simulink model "untitled"  (R2023a)
settings: Solver=VariableStepAuto  StartTime=0.0  StopTime=1  FixedStep=1e-7  MaxStep=2e-7  RelTol=1e-4
model workspace (MAT data in the model file):
  Cout = 0.00069
  Cout_esr = 0.02
  Iout_user_max = 5
  Ki_i = 800
  Ki_v = 30
  Kp_i = 0.025
  Kp_v = 0.2
  L_dcr = 0.02
  L_power = 2.2e-05
  Pout_max = 90
  Rload_extra = 8.57142857143
  Rload_heavy = 6
  Rload_light = 20
  Ts_i = 1e-05
  Ts_v = 0.0001
  Vin = 20
  Vref_max = 30
  Vref_min = 0.5
  Vset = 12
  fsw = 100000
  tdead = 2e-07
libraries: spsSeriesRLCBranchLib x4, spsMosfetLib x4, spsCurrentMeasurementLib x2, eePwmGenerator x2, spsDCVoltageSourceLib x1, spsIdealSwitchLib x1, spsMultimeterLib x1, spsVoltageMeasurementLib x1, spspowerguiLib x1
settings Model: SimulationMode=rapid-accelerator  Creator=39826  LastModifiedBy=39826

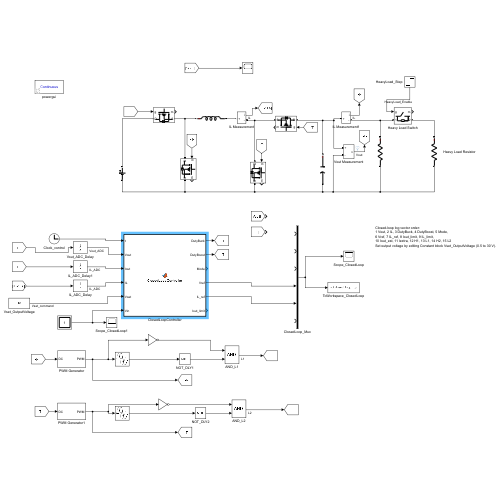
[thumbnail: Simulink's stored preview of the top-level diagram]
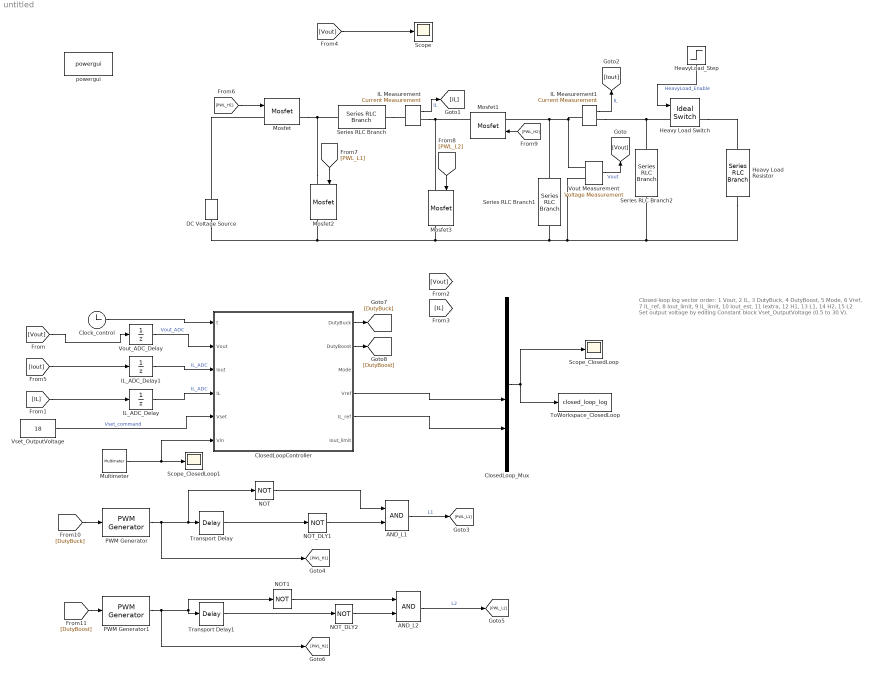
== system untitled ==
  note: Closed-loop log vector order:
      | 1 Vout, 2 IL, 3 DutyBuck, 4 DutyBoost, 5 Mode,
      | 6 Vref, 7 IL_ref, 8 Iout_limit, 9 IL_limit,
      | 10 Iout_est, 11 Iextra, 12 H1, 13 L1, 14 H2, 15 L2
      | Set output voltage by editing Constant block Vset_OutputVoltage (0.5 to 30 V).
  AND_L1 : Logic  AllPortsSameDT=off  OutDataTypeStr=boolean
  AND_L2 : Logic  AllPortsSameDT=off  OutDataTypeStr=boolean
  Clock_control : Clock
  ClosedLoopController : MATLAB Function  TreatAsAtomicUnit=on
  ClosedLoop_Mux : Mux  Inputs=6
  DC Voltage Source : spsDCVoltageSourceLib/DC Voltage Source  Amplitude=Vin  Measurements=Voltage
  Heavy Load Resistor : spsSeriesRLCBranchLib/Series RLC Branch  LConnTagsString=__new0  RConnTagsString=__new0  BranchType=R  Resistance=Rload_extra  Inductance=1e-3  SetiL0=off  InitialCurrent=0  Capacitance=1e-6  Setx0=off  InitialVoltage=0  Measurements=Branch voltage and current
  Heavy Load Switch : spsIdealSwitchLib/Ideal Switch  Ron=3e-3  Lon=0  IC=0  Rs=1e6  Cs=inf  Measurements=on
  HeavyLoad_Step : Step  SampleTime=0
  IL Measurement : spsCurrentMeasurementLib/Current Measurement  PhasorSimulation=off  OutputType=Complex  PSBequivalent=0
  IL Measurement1 : spsCurrentMeasurementLib/Current Measurement  PhasorSimulation=off  OutputType=Complex  PSBequivalent=0
  IL_ADC_Delay : UnitDelay  SampleTime=1e-6  HasFrameUpgradeWarning=on
  IL_ADC_Delay1 : UnitDelay  SampleTime=1e-6  HasFrameUpgradeWarning=on
  Mosfet{,1..3} (4 alike) : spsMosfetLib/Mosfet  Ron=3e-3  Lon=0  Rd=0.01  Vfd=0  IC=0  Rs=1e5  Cs=inf  Measurements=on
  Multimeter : spsMultimeterLib/Multimeter  L=9  sel=5  yselected={}  Gain=1  OutputType=Complex  PlotAtSimulationStop=off  PhasorSimulation=off
  NOT : Logic  Operator=NOT  IconShape=distinctive  AllPortsSameDT=off  OutDataTypeStr=boolean
  NOT1 : Logic  Operator=NOT  IconShape=distinctive  AllPortsSameDT=off  OutDataTypeStr=boolean
  NOT_DLY1 : Logic  Operator=NOT  AllPortsSameDT=off  OutDataTypeStr=boolean
  NOT_DLY2 : Logic  Operator=NOT  AllPortsSameDT=off  OutDataTypeStr=boolean
  PWM Generator : eePwmGenerator/PWM Generator  CarrCount=Up  Tper=1e-5  Tdelay=0  Ts=0
  PWM Generator1 : eePwmGenerator/PWM Generator  CarrCount=Up  Tper=1e-5  Tdelay=0  Ts=0
  Scope : Scope
  Scope_ClosedLoop : Scope
  Scope_ClosedLoop1 : Scope
  Series RLC Branch : spsSeriesRLCBranchLib/Series RLC Branch  LConnTagsString=__new0  RConnTagsString=__new0  BranchType=L  Resistance=L_dcr  Inductance=L_power  SetiL0=off  InitialCurrent=0  Capacitance=1e-6  Setx0=off  InitialVoltage=0  Measurements=Branch voltage and current
  Series RLC Branch1 : spsSeriesRLCBranchLib/Series RLC Branch  LConnTagsString=__new0  RConnTagsString=__new0  BranchType=C  Resistance=Cout_esr  Inductance=1e-3  SetiL0=off  InitialCurrent=0  Capacitance=Cout  Setx0=off  InitialVoltage=0  Measurements=Branch voltage and current
  Series RLC Branch2 : spsSeriesRLCBranchLib/Series RLC Branch  LConnTagsString=__new0  RConnTagsString=__new0  BranchType=R  Resistance=Rload_light  Inductance=1e-3  SetiL0=off  InitialCurrent=0  Capacitance=1e-6  Setx0=off  InitialVoltage=0  Measurements=Branch voltage and current
  ToWorkspace_ClosedLoop : ToWorkspace  VariableName=closed_loop_log  SaveFormat=Structure With Time  SampleTime=-1
  Transport Delay : TransportDelay  DelayTime=tdead
  Transport Delay1 : TransportDelay  DelayTime=tdead
  Vout Measurement : spsVoltageMeasurementLib/Voltage Measurement  PhasorSimulation=off  OutputType=Complex  PSBequivalent=0
  Vout_ADC_Delay : UnitDelay  SampleTime=1e-6  HasFrameUpgradeWarning=on
  Vset_OutputVoltage : Constant  Value=18
  powergui : spspowerguiLib/powergui  Priority=1  SimulationMode=Continuous  SampleTime=1e-7  frequency=60  Iterations=50  frequencyindice=0  Pbase=100e6  ErrMax=1e-4  UnitsV=kV  UnitsW=MW  buscounter=0  FunctionMessages=off  echomessages=off  EnableUseOfTLC=off  CurrentSourceSwitches=off  DisableSnubberDevices=off  DisableRonSwitches=off  DisableVfSwitches=off  DisplayEquations=off  AutomaticDiscreteSolvers=off  SolverType=Tustin/Backward Euler (TBE)  Interpol=off  ExternalGateDelay=off  methode=off  Ts=100  x0status=blocks  SPID=on  SwTol=0  HookPort=off  NonlinearTolerance=1e-4  nMaxIteration=100  ContinueOnMaxIteration=off  RestoreLinks=warning  ResistiveCurrentMeasurement=off  Frange=[0:2:500]  Ylog=off  Xlog=on  ShowGrid=off  save=off  variable=ZData  structure=0  ZoomFFT=off  StartTime=0.0  cycles=1  DisplayStyle=1  fundamental=60  FreqAxis=off  MaxFrequency=1000  frequencyindicesteady=1  RmsSteady=1  display=off
  wires:
  HeavyLoad_Step/1 -> Heavy Load Switch/1  "HeavyLoad_Enable"
  Clock_control/1 -> ClosedLoopController/1(t)
  Vout_ADC_Delay/1 -> ClosedLoopController/2(Vout)  "Vout_ADC"
  Vset_OutputVoltage/1 -> ClosedLoopController/5(Vset)  "Vset_command"
  ClosedLoop_Mux/1 -> Scope_ClosedLoop/1, ToWorkspace_ClosedLoop/1
  Vout Measurement/1 -> [Vout]  "Vout"
  [Vout] -> Vout_ADC_Delay/1
  IL Measurement/1 -> [IL]  "IL"
  [IL] -> IL_ADC_Delay/1
  [Vout] -> Scope/1
  IL_ADC_Delay/1 -> ClosedLoopController/4(IL)  "IL_ADC"
  IL Measurement1/1 -> [Iout]  "IL"
  [Iout] -> IL_ADC_Delay1/1
  IL_ADC_Delay1/1 -> ClosedLoopController/3(Iout)  "IL_ADC"
  Multimeter/1 -> Scope_ClosedLoop1/1, ClosedLoopController/6(Vin)
  PWM Generator/1 -> NOT/1, Transport Delay/1, [PWL_H1]
  PWM Generator1/1 -> NOT1/1, Transport Delay1/1, [PWL_H2]
  [PWL_H1] -> Mosfet/1
  [PWL_L1] -> Mosfet2/1
  [PWL_L2] -> Mosfet3/1
  [PWL_H2] -> Mosfet1/1
  ClosedLoopController/1(DutyBuck) -> [DutyBuck]
  ClosedLoopController/2(DutyBoost) -> [DutyBoost]
  [DutyBuck] -> PWM Generator/1
  [DutyBoost] -> PWM Generator1/1
  ClosedLoopController/5(IL_ref) -> ClosedLoop_Mux/5
  ClosedLoopController/4(Vref) -> ClosedLoop_Mux/4
  Transport Delay/1 -> NOT_DLY1/1
  NOT/1 -> AND_L1/1
  NOT_DLY1/1 -> AND_L1/2
  AND_L1/1 -> [PWL_L1]  "L1"
  Transport Delay1/1 -> NOT_DLY2/1
  NOT1/1 -> AND_L2/1
  NOT_DLY2/1 -> AND_L2/2
  AND_L2/1 -> [PWL_L2]  "L2"
  connections:
  Mosfet/LConn1 -- DC Voltage Source/RConn1
  Mosfet2/LConn1 -- Series RLC Branch/LConn1 -- Mosfet/RConn1
  Series RLC Branch/RConn1 -- IL Measurement/LConn1
  Mosfet3/LConn1 -- Mosfet1/RConn1 -- IL Measurement/RConn1
  Mosfet2/RConn1 -- DC Voltage Source/LConn1 -- Vout Measurement/LConn2 -- Heavy Load Resistor/RConn1 -- Series RLC Branch2/RConn1 -- Series RLC Branch1/RConn1 -- Mosfet3/RConn1
  Series RLC Branch2/LConn1 -- IL Measurement1/RConn1 -- Heavy Load Switch/LConn1
  Heavy Load Switch/RConn1 -- Heavy Load Resistor/LConn1
  Series RLC Branch1/LConn1 -- IL Measurement1/LConn1 -- Vout Measurement/LConn1 -- Mosfet1/LConn1

== matlab function untitled/ClosedLoopController ==
  settings: updateMethod=DISCRETE  sampleTime=Ts_i
  data: t input; Vout input; Iout input; IL input; Vset input; Vin input; DutyBuck output; DutyBoost output; Mode output; Vref output; IL_ref output; Iout_limit output; Vref_min parameter; Vref_max parameter; Iout_user_max parameter; Pout_max parameter; Ts_i parameter; Ts_v parameter; Kp_v parameter; Ki_v parameter; Kp_i parameter; Ki_i parameter
function [DutyBuck, DutyBoost, Mode, Vref, IL_ref, Iout_limit] = ClosedLoopController(t, Vout, Iout, IL, Vset, Vin, Vref_min, Vref_max, Iout_user_max, Pout_max, Ts_i, Ts_v, Kp_v, Ki_v, Kp_i, Ki_i)
%#codegen
% Ratio-based closed-loop for current model mapping: Vout ~ Vin * DutyBuck / DutyBoost
DutyBuck = 0.5;
DutyBoost = 0.5;
Mode = 2.0;
Vref = 0.0;
IL_ref = 0.0;
Iout_limit = 0.0;
small_v = 1e-3;
small_n = 1e-9;
duty_min = 0.02;
duty_max = 0.98;
kLeg = 0.96;

% 【修改 1】：引入独立的 ratioInt 变量，隔离两个通道的积分器冲突
persistent vrefRamp vInt ratioInt iInt ioutFilt ilFilt prevMode protectLatch dbPrev dsPrev vTick
if isempty(vrefRamp)
    vrefRamp = 0.0; 
    vInt = 0.0;
    ratioInt = 0.0;  % 初始化独立变比积分器
    iInt = 0.0;
    ioutFilt = 0.0;
    ilFilt = 0.0;
    prevMode = 2.0;
    protectLatch = 0.0;
    dbPrev = 0.5;
    dsPrev = 0.5;
    vTick = 0.0;
end

vout = real(Vout(1)); if ~isfinite(vout), vout = 0.0; end
iout = real(Iout(1)); if ~isfinite(iout), iout = 0.0; end
il = real(IL(1)); if ~isfinite(il), il = 0.0; end
vset = real(Vset(1)); if ~isfinite(vset), vset = 0.0; end
vin = real(Vin(1)); if ~isfinite(vin), vin = 0.0; end
vrmin = real(Vref_min(1)); if ~isfinite(vrmin), vrmin = 0.0; end
vrmax = real(Vref_max(1)); if ~isfinite(vrmax), vrmax = 30.0; end
iuser = real(Iout_user_max(1)); if ~isfinite(iuser), iuser = 0.0; end
pmax = real(Pout_max(1)); if ~isfinite(pmax), pmax = 0.0; end
tsi = real(Ts_i(1)); if ~isfinite(tsi) || tsi <= 0.0, tsi = 1e-6; end
tsv = real(Ts_v(1)); if ~isfinite(tsv) || tsv <= 0.0, tsv = tsi; end
if tsv < tsi, tsv = tsi; end
kpv = real(Kp_v(1)); if ~isfinite(kpv), kpv = 0.0; end
kiv = real(Ki_v(1)); if ~isfinite(kiv), kiv = 0.0; end
kpi = real(Kp_i(1)); if ~isfinite(kpi), kpi = 0.0; end
kii = real(Ki_i(1)); if ~isfinite(kii), kii = 0.0; end
if vrmax < vrmin
    tmp = vrmax; vrmax = vrmin; vrmin = tmp;
end
vout = max(vout, 0.0);
iout = max(iout, 0.0);
vin = max(vin, small_v);
iuser = max(iuser, 0.0);
pmax = max(pmax, 0.0);

% 【修改 2】：修复启动暴冲。启动时斜坡必须从最小值（或当前输出电压）开始，不能直接等于 vset
if t <= tsi
    vrefRamp = vrmin; % 让电压从设定的下限（例如0V或接近0V）缓缓爬升
    vInt = 0.0;
    ratioInt = 0.0;   % 重置独立变比积分器
    iInt = 0.0;
    ioutFilt = 0.0;
    ilFilt = 0.0;
    prevMode = 2.0;
    protectLatch = 0.0;
    dbPrev = 0.5;
    dsPrev = 0.5;
    vTick = 0.0;
end

% Vref clamp + ramp
vrefTar = min(max(vset, vrmin), vrmax);
% 可以根据实际需要调整下面的 3000.0（斜坡上升率，单位 V/s），觉得启动慢可以改大，觉得冲可以改小
dv = 3000.0 * tsi; 
if vrefRamp < vrefTar
    vrefRamp = min(vrefRamp + dv, vrefTar);
else
    vrefRamp = max(vrefRamp - dv, vrefTar);
end
Vref = min(max(vrefRamp, vrmin), vrmax);

% Current/power limit requirement
Iout_limit = min(iuser, pmax / max(vout, small_v));
Iout_limit = max(Iout_limit, 0.0);

% Filters
ioutFilt = 0.9 * ioutFilt + 0.1 * iout;
ilFilt = 0.9 * ilFilt + 0.1 * il;

% Mode selection with hysteresis
ratioFF = Vref / max(vin, small_v);
if prevMode < 1.0 || prevMode > 4.0
    prevMode = 2.0;
end
if prevMode == 1.0
    if ratioFF > 0.98, modeSel = 2.0; else, modeSel = 1.0; end
elseif prevMode == 3.0
    if ratioFF < 1.02, modeSel = 2.0; else, modeSel = 3.0; end
else
    if ratioFF < 0.95, modeSel = 1.0;
    elseif ratioFF > 1.05, modeSel = 3.0;
    else, modeSel = 2.0;
    end
end

% Severe over-current latch
tripI = max(1.8 * Iout_limit, 0.2);
relI = max(0.9 * Iout_limit, 0.1);
if protectLatch < 0.5
    if ioutFilt > tripI, protectLatch = 1.0; end
else
    if ioutFilt < relI, protectLatch = 0.0; end
end
if protectLatch >= 0.5
    Mode = 4.0;
else
    Mode = modeSel;
end
if Mode ~= prevMode
    iInt = 0.0;
    prevMode = Mode;
end

% Cascaded structure outputs
ilLimit = min(max(1.25 * Iout_limit * max(Vref, vin) / max(vin, small_v), 0.1), 25.0);
vTick = vTick + tsi;
if vTick >= tsv
    vTick = vTick - tsv;
    eV = Vref - vout;
    vCand = vInt + kiv * tsv * eV;
    ilUnsat = kpv * eV + vCand;
    atHigh = (ilUnsat >= ilLimit) && (eV > 0.0);
    atLow = (ilUnsat <= 0.0) && (eV < 0.0);
    if ~(atHigh || atLow)
        vInt = vCand; % 此处 vInt 纯净地留给外环级联使用
    end
end
IL_ref = min(max(kpv * (Vref - vout) + vInt, 0.0), ilLimit);

% Inner loop as correction term
eI = IL_ref - ilFilt;
iCand = iInt + kii * tsi * eI;
rawIcorr = kpi * eI + iCand;
icorrSat = min(max(rawIcorr, -0.08), 0.08);
if (abs(rawIcorr - icorrSat) < 1e-12) || (sign(eI) ~= sign(rawIcorr - icorrSat))
    iInt = iCand;
end

% Direct voltage PI on ratio
KvP = max(0.05 * kpv, 0.01);
KvI = max(0.10 * kiv, 1.0);
ratioErr = Vref - vout;

% 【修改 3】：改用独立的 ratioInt，彻底切断与串级外环 vInt 的冲突拉扯
ratioIntCand = ratioInt + KvI * tsi * ratioErr; 
ratioRaw = ratioFF + KvP * ratioErr + ratioIntCand + 0.2 * icorrSat;
ratioMin = duty_min / duty_max;
ratioMax = duty_max / duty_min;
ratioCmd = min(max(ratioRaw, ratioMin), ratioMax);

% 对主通道独立的积分器进行抗饱和限制
ratioSatHigh = (ratioRaw >= ratioMax) && (ratioErr > 0.0);
ratioSatLow = (ratioRaw <= ratioMin) && (ratioErr < 0.0);
if ~(ratioSatHigh || ratioSatLow)
    ratioInt = ratioIntCand; 
end

% Duty synthesis from ratio command
if ratioCmd >= 1.0
    dbRef = kLeg;
    dsRef = kLeg / ratioCmd;
else
    dsRef = kLeg;
    dbRef = kLeg * ratioCmd;
end

% Mode-specific slight bias 
% 【优化提示】：如果发现稳态纹波依然存在，可以尝试将下面的 0.01 改为 0（彻底移除模式切换死区阶跃）
if Mode == 1.0
    dsRef = min(max(dsRef + 0.01, duty_min), duty_max);
elseif Mode == 3.0
    dbRef = min(max(dbRef + 0.01, duty_min), duty_max);
elseif Mode == 4.0
    dbRef = duty_min;
    dsRef = duty_max;
    IL_ref = 0.0;
end
dbRef = min(max(dbRef, duty_min), duty_max);
dsRef = min(max(dsRef, duty_min), duty_max);

% Slew-rate limit to reduce jitter/ripple
slew = 0.01;
DutyBuck = dbPrev + min(max(dbRef - dbPrev, -slew), slew);
DutyBoost = dsPrev + min(max(dsRef - dsPrev, -slew), slew);
DutyBuck = min(max(DutyBuck, duty_min), duty_max);
DutyBoost = min(max(DutyBoost, duty_min), duty_max);

% Extra pull-down if over output current limit
if Iout_limit > small_n && ioutFilt > Iout_limit
    kOver = min(max((ioutFilt / Iout_limit - 1.0), 0.0), 1.0);
    DutyBuck = max(duty_min, DutyBuck - 0.05 * kOver);
    DutyBoost = min(duty_max, DutyBoost + 0.05 * kOver);
end
dbPrev = DutyBuck;
dsPrev = DutyBoost;
end
